simulink model "Glider"  (R2017b)
settings: Solver=ode4  StartTime=0.0  StopTime=200.0  FixedStep=0.1  RelTol=1e-3
libraries: simulink x1
settings Model: Creator=whsteyn  LastModifiedBy=whsteyn
settings DataIOCC: LimitDataPoints=on  SaveFormat=Array  SignalLoggingSaveFormat=ModelDataLogs
settings OptimizationCC: InitFltsAndDblsToZero=on  LifeSpan=inf
settings DebuggingCC: SaveWithParameterizedLinksMsg=none  UnderspecifiedInitializationDetection=Classic  MergeDetectMultiDrivingBlocksExec=none  SignalResolutionControl=TryResolveAllWithWarning  SolverPrmCheckMsg=warning  MultiTaskDSMMsg=warning  MultiTaskCondExecSysMsg=none  FcnCallInpInsideContextMsg=warning  SFUnexpectedBacktrackingDiag=warning  SFNoUnconditionalDefaultTransitionDiag=warning  SFExecutionAtInitializationDiag=none
settings HardwareCC: ProdBitPerPointer=32  ProdBitPerSizeT=32  ProdBitPerPtrDiffT=32  ProdLargestAtomicFloat=None  ProdIntDivRoundTo=Undefined  ProdEndianess=Unspecified  ProdWordSize=32  ProdHWDeviceType=32-bit Generic
settings ModelReferenceCC: PropagateSignalLabelsOutOfModel=off
settings CodeAppCC: StateflowObjectComments=on
settings GRTTargetCC: TargetFcnLib=ansi_tfl_tmw.mat  TargetLangStandard=C89/C90 (ANSI)  GeneratePreprocessorConditionals=Disable all  CombineOutputUpdateFcns=off  GRTInterface=on
settings ConfigComp: CovMetricSettings=dw  CovHtmlReporting=on  CovSaveCumulativeToWorkspaceVar=on  CovSaveSingleToWorkspaceVar=on  CovExternalEMLEnable=off  CovSFcnEnable=off

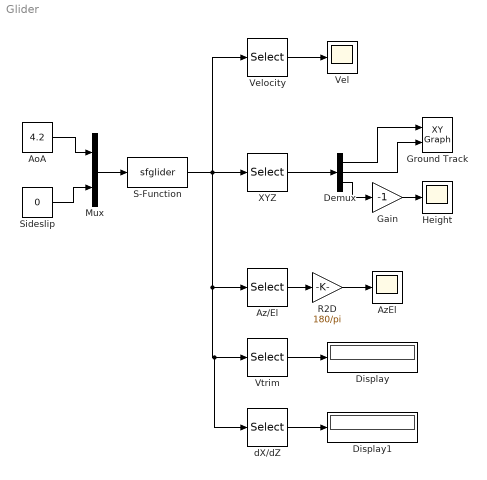
== system Glider ==
  AoA : Constant  Value=4.2
  Az/El : Selector  InputPortWidth=8  IndexOptions=Index vector (dialog)  Indices=[5,6]  OutputSizes=1
  AzEl : Scope
  Demux : Demux  Outputs=3
  Display : Display
  Display1 : Display
  Gain : Gain  Gain=-1
  Ground Track : simulink/Sinks/XY Graph  xmin=0  xmax=2500  ymin=-1000  ymax=1000  st=-1
  Height : Scope
  Mux : Mux  Inputs=2
  R2D : Gain  Gain=180/pi
  S-Function : S-Function  FunctionName=sfglider  Parameters=11.25,1000,2.5,[0 -2.74 0]  SFunctionDeploymentMode=off  EnableBusSupport=off
  Sideslip : Constant  Value=0
  Vel : Scope
  Velocity : Selector  InputPortWidth=8  IndexOptions=Index vector (dialog)  Indices=[4]  OutputSizes=1
  Vtrim : Selector  InputPortWidth=8  IndexOptions=Index vector (dialog)  Indices=[7]  OutputSizes=1
  XYZ : Selector  InputPortWidth=8  IndexOptions=Index vector (dialog)  Indices=[1:3]  OutputSizes=1
  dX/dZ : Selector  InputPortWidth=8  IndexOptions=Index vector (dialog)  Indices=[8]  OutputSizes=1
  wires:
  Mux/1 -> S-Function/1
  S-Function/1 -> Velocity/1, XYZ/1, dX/dZ/1, Vtrim/1, Az/El/1
  XYZ/1 -> Demux/1
  Velocity/1 -> Vel/1
  AoA/1 -> Mux/1
  Gain/1 -> Height/1
  Demux/3 -> Gain/1
  Demux/1 -> Ground Track/1
  Demux/2 -> Ground Track/2
  Sideslip/1 -> Mux/2
  Az/El/1 -> R2D/1
  R2D/1 -> AzEl/1
  Vtrim/1 -> Display/1
  dX/dZ/1 -> Display1/1
